simulink model "simulink_control_effort_step"  (R2022b)
settings: Solver=VariableStepAuto  StartTime=0.0  StopTime=10.0  RelTol=1e-3
settings Model: Creator=MSH8303  LastModifiedBy=MSH8303

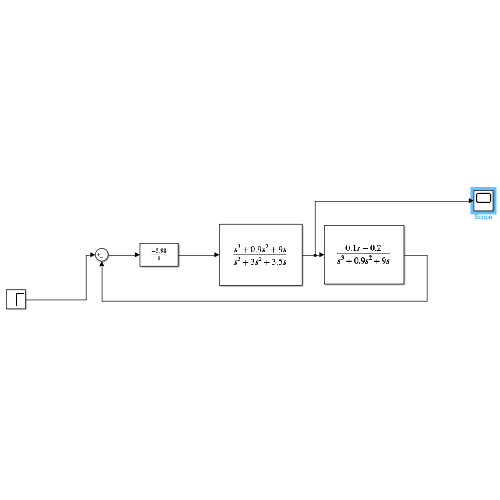
[thumbnail: Simulink's stored preview of the top-level diagram]
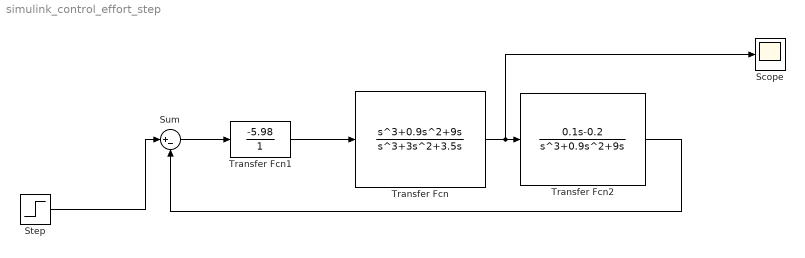
== system simulink_control_effort_step ==
  Scope : Scope
  Step : Step  SampleTime=0
  Sum : Sum  Inputs=|+-
  Transfer Fcn : TransferFcn  Numerator=[1 0.9 9 0]  Denominator=[1 3 3.5 0]
  Transfer Fcn1 : TransferFcn  Numerator=[-5.98]  Denominator=[1]
  Transfer Fcn2 : TransferFcn  Numerator=[0.1 -0.2]  Denominator=[1 0.9 9 0]
  wires:
  Sum/1 -> Transfer Fcn1/1
  Transfer Fcn1/1 -> Transfer Fcn/1
  Transfer Fcn/1 -> Scope/1, Transfer Fcn2/1
  Transfer Fcn2/1 -> Sum/2
  Step/1 -> Sum/1
